simulink model "Simulation_1"  (R2018a)
settings: Solver=VariableStepAuto  StartTime=0.0  StopTime=100e-3  MaxStep=1e-6  RelTol=1e-5
libraries: powerlib x11, simulink x1
settings Model: Creator=mahadi  LastModifiedBy=mahadi
settings SolverCC: InitialStep=1e-6

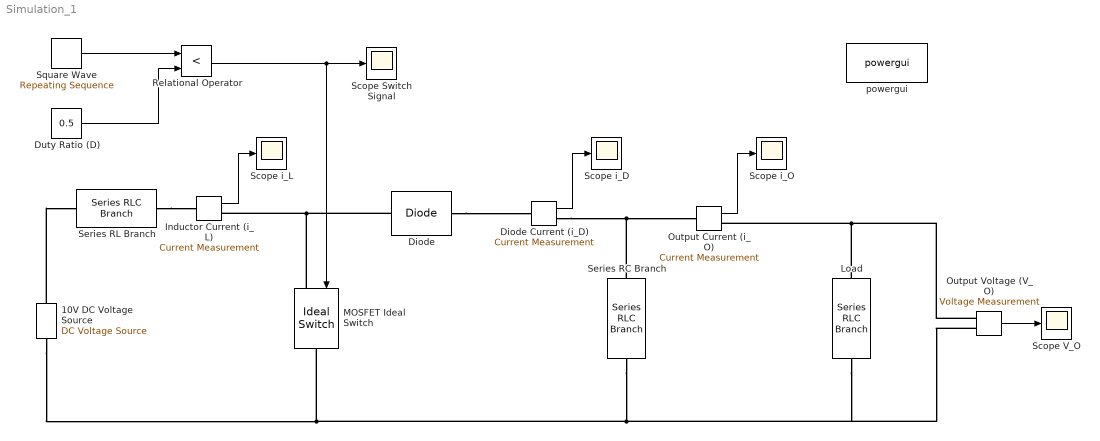
== system Simulation_1 ==
  " 10V DC Voltage Source" : powerlib/Electrical Sources/DC Voltage Source  Amplitude=10  Measurements=Voltage
  "Diode " : powerlib/Power Electronics/Diode  Ron=0.01  Lon=0  Vf=0.8  IC=0  UseSnubber=0  Rs=1e5  Cs=250e-9  Measurements=off
  Diode Current (i_D) : powerlib/Measurements/Current Measurement  PhasorSimulation=off  OutputType=Complex  PSBequivalent=0
  Duty Ratio (D) : Constant  Value=0.5
  Inductor Current (i_L) : powerlib/Measurements/Current Measurement  PhasorSimulation=off  OutputType=Complex  PSBequivalent=0
  Load : powerlib/Elements/Series RLC Branch  LConnTagsString=__new0  RConnTagsString=__new0  BranchType=R  Resistance=470  Inductance=1e-3  SetiL0=off  InitialCurrent=0  Capacitance=100e-6  Setx0=off  InitialVoltage=0  Measurements=None
  MOSFET Ideal Switch : powerlib/Power Electronics/Ideal Switch  Ron=0.01  Lon=0  IC=0  Rs=1e10  Cs=inf  Measurements=off
  Output Current (i_O) : powerlib/Measurements/Current Measurement  PhasorSimulation=off  OutputType=Complex  PSBequivalent=0
  Output Voltage (V_O) : powerlib/Measurements/Voltage Measurement  PhasorSimulation=off  OutputType=Complex  PSBequivalent=0
  "Relational Operator " : RelationalOperator  Operator=<  OutDataTypeStr=boolean  RndMeth=Simplest
  Scope Switch Signal : Scope
  Scope V_O : Scope
  Scope i_D : Scope
  Scope i_L : Scope
  Scope i_O : Scope
  Series RC Branch : powerlib/Elements/Series RLC Branch  LConnTagsString=__new0  RConnTagsString=__new0  BranchType=RC  Resistance=20e-3  Inductance=1e-3  SetiL0=off  InitialCurrent=0  Capacitance=100e-6  Setx0=off  InitialVoltage=0  Measurements=None
  Series RL Branch : powerlib/Elements/Series RLC Branch  LConnTagsString=__new0  RConnTagsString=__new0  BranchType=RL  Resistance=1  Inductance=10e-3  SetiL0=off  InitialCurrent=0  Capacitance=1e-6  Setx0=off  InitialVoltage=0  Measurements=None
  Square Wave : simulink/Sources/Repeating Sequence  rep_seq_t=[0 1e-4]  rep_seq_y=[0 1]
  "powergui " : powerlib/powergui  Priority=1  SimulationMode=Continuous  SampleTime=50e-6  frequency=60  Iterations=50  frequencyindice=0  Pbase=100e6  ErrMax=1e-4  UnitsV=kV  UnitsW=MW  buscounter=0  FunctionMessages=off  echomessages=off  EnableUseOfTLC=off  CurrentSourceSwitches=off  DisableSnubberDevices=off  DisableRonSwitches=off  DisableVfSwitches=off  DisplayEquations=off  SolverType=Tustin/Backward Euler (TBE)  Interpol=off  ExternalGateDelay=off  methode=off  Ts=100  x0status=blocks  SPID=on  SwTol=0  HookPort=off  RestoreLinks=warning  ResistiveCurrentMeasurement=off  Frange=[0:2:500]  Ylog=off  Xlog=on  ShowGrid=off  save=off  variable=ZData  structure=0  ZoomFFT=off  StartTime=0.0  cycles=1  DisplayStyle=1  fundamental=60  FreqAxis=off  MaxFrequency=1000  frequencyindicesteady=1  RmsSteady=1  display=off
  wires:
  Output Voltage (V_O)/1 -> Scope V_O/1
  Diode Current (i_D)/1 -> Scope i_D/1
  Output Current (i_O)/1 -> Scope i_O/1
  Square Wave/1 -> "Relational Operator "/1
  Duty Ratio (D)/1 -> "Relational Operator "/2
  "Relational Operator "/1 -> MOSFET Ideal Switch/1, Scope Switch Signal/1
  Inductor Current (i_L)/1 -> Scope i_L/1
  connections:
  " 10V DC Voltage Source"/RConn1 -- Series RL Branch/LConn1
  Series RL Branch/RConn1 -- Inductor Current (i_L)/LConn1
  "Diode "/LConn1 -- MOSFET Ideal Switch/LConn1 -- Inductor Current (i_L)/RConn1
  " 10V DC Voltage Source"/LConn1 -- Load/RConn1 -- Output Voltage (V_O)/LConn2 -- Series RC Branch/RConn1 -- MOSFET Ideal Switch/RConn1
  "Diode "/RConn1 -- Diode Current (i_D)/LConn1
  Diode Current (i_D)/RConn1 -- Series RC Branch/LConn1 -- Output Current (i_O)/LConn1
  Output Voltage (V_O)/LConn1 -- Load/LConn1 -- Output Current (i_O)/RConn1
